simulink model "Helicopter_Non_linear_Original"  (R2018a)
settings: Solver=ode4  StartTime=0.0  StopTime=inf  FixedStep=0.2  RelTol=1e-3
values from neighbouring files (symbols this model uses):
  Bp = 0.01    [Helicopter_Values.m]
  By = 0.08    [Helicopter_Values.m]
  g = 9.81    [Helicopter_Values.m]
  jeqp = 0.0172    [Helicopter_Values.m]
  jeqy = 0.021    [Helicopter_Values.m]
  kpp = 0.0556    [Helicopter_Values.m]
  kpy = 0.005    [Helicopter_Values.m]
  kyp = 0.15    [Helicopter_Values.m]
  kyy = 0.21084    [Helicopter_Values.m]
  lcm = 0.015    [Helicopter_Values.m]
  mheli = 0.479    [Helicopter_Values.m]
undefined symbols (not defined in the file or in its folder): d2r
libraries: realtime_pacer_lib x1
settings Model: Creator=pacoa  LastModifiedBy=pacoa

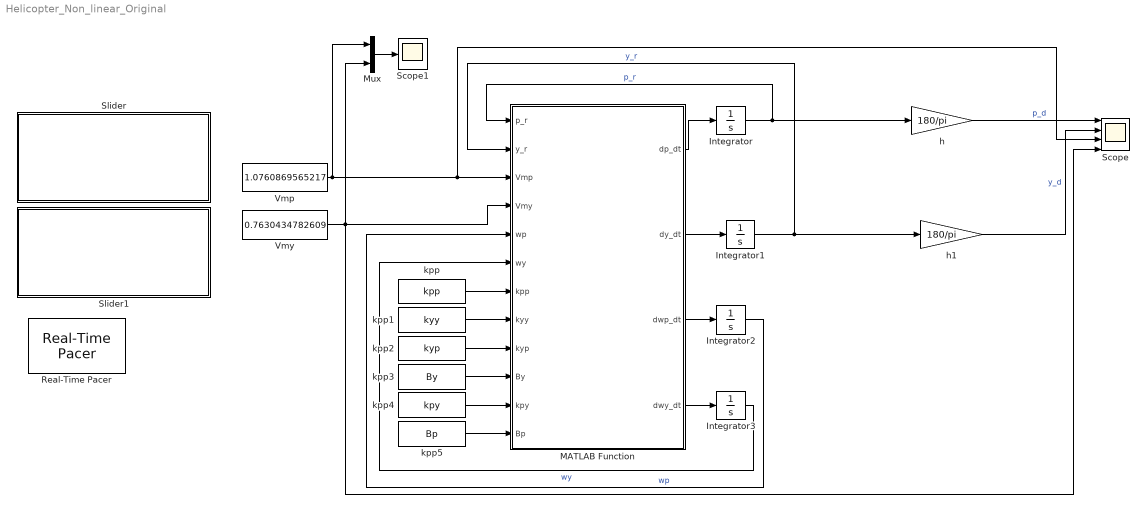
== system Helicopter_Non_linear_Original ==
  Integrator : Integrator  InitialCondition=d2r(-31.0537918783631)  LimitOutput=on  UpperSaturationLimit=pi/4  LowerSaturationLimit=-pi/4
  Integrator1 : Integrator  InitialCondition=d2r(120.519928781055)  LimitOutput=on  UpperSaturationLimit=pi  LowerSaturationLimit=0
  Integrator2 : Integrator  UpperSaturationLimit=1  LowerSaturationLimit=-1
  Integrator3 : Integrator
  MATLAB Function : MATLAB Function  TreatAsAtomicUnit=on
  Mux : Mux  Inputs=2
  Real-Time Pacer : realtime_pacer_lib/Real-Time Pacer  simTimePerRealTime=10
  Scope : Scope  NumInputPorts=4
  Scope1 : Scope
  Slider : Subsystem  DialogController=hmiCreateDDGDialog  IsWebBlock=on  mask(MWDashboardBlock){webBlockId=66175977-3272-42b5-ab67-6b4a8954cffe, webBlockType=slider, ShowInLibBrowser=on, ShowInitialText=on, HMISrcModelName=Helicopter_Non_linear_Original}
      mask prompts: webBlockId "WebBlock Id"; webBlockType "WebBlock Type"; HMISrcModelName "Source Model"
      mask help: SimulinkHMI:dialogs:SliderDialogDesc
      mask Help: helpview([docroot '/mapfiles/simulink.map'], 'hmi_slider')
      mask Display:
      | if strcmp(get_param(bdroot(gcb),'BlockDiagramType'), 'library')
      |     image([(matlabroot) '/toolbox/simulink/hmi/icons/Slider.png']);
      | end
  Slider1 : Subsystem  DialogController=hmiCreateDDGDialog  IsWebBlock=on  mask(MWDashboardBlock){webBlockId=07336fed-dc62-42af-98e1-995325230895, webBlockType=slider, ShowInLibBrowser=on, ShowInitialText=on, HMISrcModelName=Helicopter_Non_linear_Original}
      mask prompts: webBlockId "WebBlock Id"; webBlockType "WebBlock Type"; HMISrcModelName "Source Model"
      mask help: SimulinkHMI:dialogs:SliderDialogDesc
      mask Help: helpview([docroot '/mapfiles/simulink.map'], 'hmi_slider')
      mask Display:
      | if strcmp(get_param(bdroot(gcb),'BlockDiagramType'), 'library')
      |     image([(matlabroot) '/toolbox/simulink/hmi/icons/Slider.png']);
      | end
  Vmp : Constant  Value=1.0760869565217
  Vmy : Constant  Value=0.7630434782609
  h : Gain  Gain=180/pi
  h1 : Gain  Gain=180/pi
  kpp : Constant  Value=kpp
  kpp1 : Constant  Value=kyy
  kpp2 : Constant  Value=kyp
  kpp3 : Constant  Value=By
  kpp4 : Constant  Value=kpy
  kpp5 : Constant  Value=Bp
  wires:
  kpp2/1 -> MATLAB Function/9(kyp)
  kpp3/1 -> MATLAB Function/10(By)
  kpp5/1 -> MATLAB Function/12(Bp)
  MATLAB Function/1(dp_dt) -> Integrator/1
  MATLAB Function/3(dwp_dt) -> Integrator2/1
  kpp4/1 -> MATLAB Function/11(kpy)
  Vmy/1 -> Scope/4, Mux/2, MATLAB Function/4(Vmy)
  kpp/1 -> MATLAB Function/7(kpp)
  Integrator1/1 -> MATLAB Function/2(y_r), h1/1  "y_r"
  MATLAB Function/2(dy_dt) -> Integrator1/1
  Integrator3/1 -> MATLAB Function/6(wy)  "wy"
  h/1 -> Scope/1  "p_d"
  h1/1 -> Scope/2  "y_d"
  Integrator2/1 -> MATLAB Function/5(wp)  "wp"
  Vmp/1 -> Mux/1, MATLAB Function/3(Vmp), Scope/3
  Integrator/1 -> h/1, MATLAB Function/1(p_r)  "p_r"
  kpp1/1 -> MATLAB Function/8(kyy)
  MATLAB Function/4(dwy_dt) -> Integrator3/1
  Mux/1 -> Scope1/1

== system Helicopter_Non_linear_Original/Slider ==

== system Helicopter_Non_linear_Original/Slider1 ==

== matlab function Helicopter_Non_linear_Original/MATLAB Function ==
  data: p_r input; y_r input; Vmp input; Vmy input; wp input; dp_dt output size=[1 1]; wy input; dy_dt output size=[1 1]; dwp_dt output size=[1 1]; dwy_dt output size=[1 1]; lcm parameter; mheli parameter; jeqp parameter; jeqy parameter; g parameter; kpp input; kyy input; kyp input; By input; kpy input; Bp input
function [dp_dt, dy_dt, dwp_dt, dwy_dt]= fcn(p_r,y_r,Vmp, Vmy,wp,wy, lcm, mheli, jeqp, jeqy, g, kpp, kyy, kyp, By, kpy, Bp)

  %%Parameters
%   
%   Bp,
%   By,
%   g,
%   kpp,
%   kyp,
%   kyy,
%   kpy,
%   mheli,
%   lcm,
%   jeqp,
%   jeqy,
  

%%
   dp_dt = wp;
   dy_dt = wy;
   
   %%
   dwp_dt_n1 = (kpp*Vmp);
   dwp_dt_n2 = (kpy*Vmy);
   dwp_dt_n3 = (Bp*wp+ (mheli*(wy.^2)*sin(p_r)*(lcm^2)*cos(p_r) + (mheli*g*cos(p_r)*lcm)));
   
   dwp_dt_d = (jeqp + mheli*(lcm^2));
   
   dwp_dt = (dwp_dt_n1 -dwp_dt_n2 - dwp_dt_n3)/(dwp_dt_d);
   
   %%
   dwy_dt_n1 = kyp*Vmp;
   dwy_dt_n2 = kyy*Vmy;
   dwy_dt_n3 = 2*mheli*(wy)*sin(p_r)*(lcm^2)*cos(p_r)*wp;
   dwy_dt_n4 = By*wy;
   
   dwy_dt_d = jeqy + mheli*((cos(p_r))^2)*(lcm^2);
   
   dwy_dt = (dwy_dt_n1 - dwy_dt_n2 + dwy_dt_n3 -dwy_dt_n4)/(dwy_dt_d);
